simulink model "ekfpromax"  (R2025b)
settings: Solver=VariableStepAuto  StartTime=0.0  StopTime=10.0  RelTol=1e-3
settings Model: Creator=fouca  LastModifiedBy=fouca

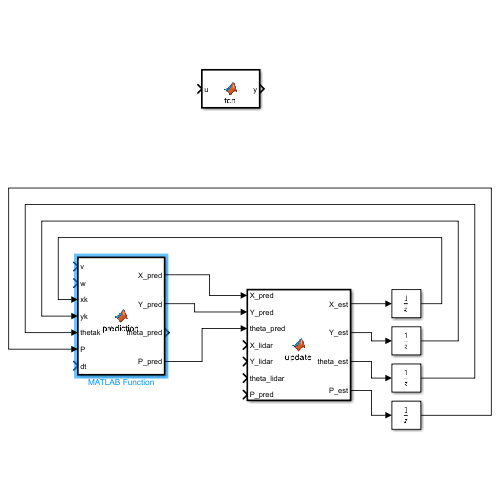
[thumbnail: Simulink's stored preview of the top-level diagram]
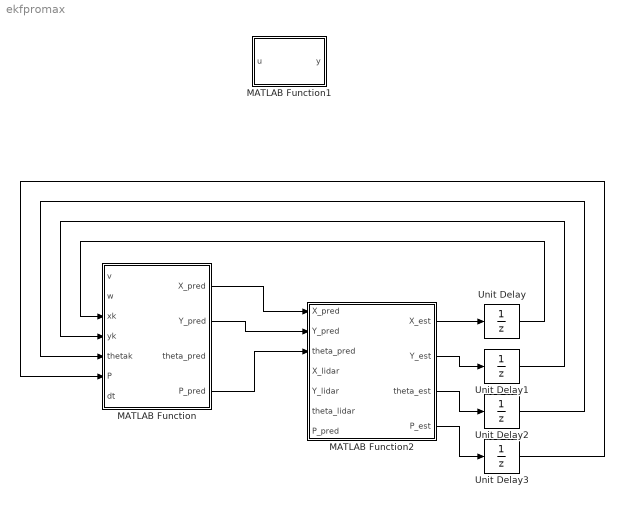
== system ekfpromax ==
  MATLAB Function : MATLAB Function  TreatAsAtomicUnit=on
  MATLAB Function1 : MATLAB Function  TreatAsAtomicUnit=on
  MATLAB Function2 : MATLAB Function  TreatAsAtomicUnit=on
  Unit Delay{,1..3} (4 alike) : UnitDelay  SampleTime=-1  HasFrameUpgradeWarning=on
  wires:
  MATLAB Function/1(X_pred) -> MATLAB Function2/1(X_pred)
  MATLAB Function/2(Y_pred) -> MATLAB Function2/2(Y_pred)
  MATLAB Function/4(P_pred) -> MATLAB Function2/3(theta_pred)
  MATLAB Function2/1(X_est) -> Unit Delay/1
  Unit Delay/1 -> MATLAB Function/3(xk)
  Unit Delay1/1 -> MATLAB Function/4(yk)
  MATLAB Function2/2(Y_est) -> Unit Delay1/1
  MATLAB Function2/3(theta_est) -> Unit Delay2/1
  Unit Delay2/1 -> MATLAB Function/5(thetak)
  MATLAB Function2/4(P_est) -> Unit Delay3/1
  Unit Delay3/1 -> MATLAB Function/6(P)

== matlab function ekfpromax/MATLAB Function1 ==
  data: u input; y output
function y = fcn(u)

y = u;

== matlab function ekfpromax/MATLAB Function ==
  data: v input; X_pred output; Y_pred output; theta_pred output; w input; P_pred output; xk input; yk input; thetak input; P input; dt input
function [X_pred, Y_pred, theta_pred, P_pred] = prediction(v, w, xk, yk, thetak, P, dt)
    % Vecteur d'état actuel
    X = [xk; yk; thetak];
    
    % 1. MODÈLE D'ÉTAT (Cinématique du QBot)
    % On calcule la prédiction basée sur les vitesses v (linéaire) et w (angulaire)
    X_next = X + [v * cos(thetak) * dt;
                  v * sin(thetak) * dt;
                  w * dt];
    
    % Extraction des sorties individuelles pour ton schéma
    X_pred     = X_next(1);
    Y_pred     = X_next(2);
    theta_pred = atan2(sin(X_next(3)), cos(X_next(3))); % Normalisation d'angle (-pi à pi)

    % 2. LINÉARISATION (Calcul de la Jacobienne F)
    % f est la dérivée de l'équation d'état par rapport à x, y et theta
    F = [1, 0, -v * sin(thetak) * dt;
         0, 1,  v * cos(thetak) * dt;
         0, 0,  1];

    % 3. BRUIT DE MODÈLE (Matrice Q)
    % Plus ces valeurs sont élevées, moins on fait confiance au modèle théorique
    % À ajuster selon les glissements des roues du QBot
    q_x = 0.01; 
    q_y = 0.01;
    q_theta = 0.02;
    Q = diag([q_x, q_y, q_theta]);

    % 4. PRÉDICTION DE LA COVARIANCE
    % On propage l'incertitude P_pred = F*P*F' + Q
    P_pred = F * P * F' + Q;
end

== matlab function ekfpromax/MATLAB Function2 ==
  data: X_pred input; X_est output; Y_pred input; theta_pred input; X_lidar input; Y_lidar input; theta_lidar input; Y_est output; theta_est output; P_est output; P_pred input
function [X_est, Y_est, theta_est, P_est] = update(X_pred, Y_pred, theta_pred, X_lidar, Y_lidar, theta_lidar, P_pred)
    % 1. VECTEURS D'ÉTAT ET DE MESURE
    x_p = [X_pred; Y_pred; theta_pred];
    z = [X_lidar; Y_lidar; theta_lidar];
    
    % 2. MODÈLE D'OBSERVATION (H)
    % Puisque le LIDAR mesure directement x, y et theta, H est l'identité
    H = eye(3);
    
    % 3. MATRICE DE BRUIT DE MESURE (R)
    % Plus ces valeurs sont faibles, plus le filtre fera confiance au LIDAR
    % (À ajuster selon la précision de votre LIDAR)
    r_dist = 0.05; % Incertitude en mètres
    r_ang  = 0.02; % Incertitude en radians
    R = diag([r_dist, r_dist, r_ang]);
    
    % 4. CALCUL DU GAIN DE KALMAN (K)
    % S est la covariance de l'innovation
    S = H * P_pred * H' + R;
    K = P_pred * H' / S;
    
    % 5. CALCUL DE L'INNOVATION (Erreur entre LIDAR et Prédiction)
    innovation = z - (H * x_p);
    
    % --- TRÈS IMPORTANT : Normalisation de l'erreur d'angle ---
    % Empêche le filtre de paniquer si le LIDAR dit 179° et le modèle 181° (-179°)
    innovation(3) = atan2(sin(innovation(3)), cos(innovation(3)));
    
    % 6. MISE À JOUR DE L'ÉTAT ET DE LA COVARIANCE
    x_corrected = x_p + K * innovation;
    P_corrected = (eye(3) - K * H) * P_pred;
    
    % 7. ASSIGNATION DES SORTIES
    X_est = x_corrected(1);
    Y_est = x_corrected(2);
    theta_est = atan2(sin(x_corrected(3)), cos(x_corrected(3)));
    P_est = P_corrected;
end
